simulink model "ADAS_Main_ClosedLoop"  (R2026a)
settings: Solver=FixedStepDiscrete  StopTime=20
InitFcn:
  | createLidarActorProfiles;
  | % L3/L4 closed-loop ego initial condition, READ FROM THE TEST-1 FIXTURE
  | % (not hard-coded in the vehicle model, which stays reusable)
  | clS = load('D:\AutonomousDriving\D_scenarios\V2_0_ClosedLoop_Test9_TwoObstacles_WideRoad.mat');
  | clA = clS.data.ActorSpecifications([clS.data.ActorSpecifications.ActorID] == clS.data.EgoCarId);
  | CL_EGO_IC = [clA.Position(1); clA.Position(2); clA.Yaw*pi/180; clA.Speed(1)];
  | clear clS clA
  | % Non-virtual ego-pose bus type. A MATLAB Function block (Extract_Ego_Kinematics)
  | % cannot accept a VIRTUAL bus, so the Bus Creator must emit a defined Simulink.Bus.
  | % Shape copied from the installed validator contract and from BusActorsActors.
  | clN = {'ActorID','Position','Velocity','Roll','Pitch','Yaw','AngularVelocity'};
  | clD = {[1 1],[1 3],[1 3],[1 1],[1 1],[1 1],[1 3]};
  | clEls = Simulink.BusElement.empty(0,1);
  | for clI = 1:7
  |   clE = Simulink.BusElement; clE.Name = clN{clI}; clE.Dimensions = clD{clI}; clE.DataType = 'double';
  |   clEls(clI,1) = clE;
  | end
  | BusEgoPose_CL = Simulink.Bus; BusEgoPose_CL.Elements = clEls;
  | clear clN clD clEls clE clI
StopFcn:
  | cl_plot_closedloop_trajectory;
model workspace (MAT data in the model file):
  firstWarning = 1
  originalScenarioChecksum = '71EAF3DF157DF5A35F75811B676F8B0F'
undefined symbols (not defined in the file): driving, matlabshared
libraries: drivingscenarioandsensors x3, lidarlib x1
(part 7 of 7)

== matlab function ADAS_Main_ClosedLoop/LiDAR_Perception/LiDAR_Ground_Segmentation/Ground_Height_Model ==
  data: xyzEgo input; groundZ output; groundMask input; groundZValid output
function [groundZ, groundZValid] = Ground_Height_Model(xyzEgo, groundMask)
%#codegen
% GROUND_HEIGHT_MODEL  Compact polar ground-elevation map from LiDAR ground returns.
%
% Inputs
%   xyzEgo     [101 2251 3] double  organized XYZ in the EGO frame
%   groundMask [101 2251]   boolean ground cells from Ground_Segmentation
%                                   (already a subset of the valid mask)
% Outputs
%   groundZ      [72 24] double   ego-frame z of the road surface, metres
%   groundZValid [72 24] boolean  true only where groundZ is a real measurement
%
% COORDINATE FRAME
%   Ego / vehicle frame: origin at the rear-axle centre, X forward, Y left,
%   Z up - the same frame Radar and Vision report in. Cells are indexed by
%   ego-frame polar coordinates about the ego origin:
%       r     = hypot(x,y)          azimuth = atan2(y,x) wrapped to (-pi,pi]
%   so a downstream lookup by an object's own ego-frame range/azimuth is
%   self-consistent with this binning.
%
% BINNING
%   Azimuth: N_AZ uniform sectors over 360 deg.
%   Range:   N_RNG GEOMETRIC (log-spaced) bins over [RMIN, RMAX].
%   Log spacing is dictated by sensor geometry, not by any scenario: the
%   radial gap between consecutive ground hits grows as r^2*dPhi/h, so ground
%   sample density falls as r^2. Uniform rings would put nearly every sample
%   in the first ring. RMAX is the sensor's MaxRange, deliberately NOT tuned
%   to the ground extent of any particular scene; unobserved cells simply
%   report invalid.
%
% ESTIMATION
%   Per cell, the median of stride-sampled ego-frame z values. Stride sampling
%   (rather than first-K) keeps the sample unbiased across the cell instead of
%   favouring one elevation row. The median is robust to the small fraction of
%   mislabelled ground points.
%
% VALIDITY  (groundZValid)
%   1. support : at least MIN_GROUND_PTS_PER_CELL samples in the cell
%   2. flatness: interquartile spread <= MAX_GROUND_SPREAD
%   3. radial slope continuity: walking outward along each azimuth sector, the
%      seed ring must satisfy |z| <= MAX_SLOPE*r + SLOPE_EPS (the ego frame
%      origin sits at ground level, and road grade is physically bounded), and
%      every subsequent accepted ring must be reachable from the previous one
%      at no more than MAX_SLOPE. This rejects flat elevated surfaces - for
%      example a neighbouring vehicle roof - that survive tests 1 and 2.
%
% MISSING REGIONS
%   Where validity fails, groundZ is set to 0 as a NUMERIC PLACEHOLDER ONLY.
%   It is not a measurement and must never be used as one. There is NO
%   interpolation and NO neighbour fallback in this stage: groundZValid means
%   exactly "measured in this cell". Any fallback policy belongs downstream,
%   where it can raise its own observation flag.
%
% SCENARIO INDEPENDENCE
%   Consumes only geometry and the ground mask. No ActorID, ClassID,
%   MaterialID, cluster metadata, actor poses, actor profiles or road geometry.

% ---- parameters: sensor / algorithm / road-physics properties only --------
N_AZ       = 72;      % azimuth sectors (5 deg each)
N_RNG      = 24;      % geometric range bins
RMIN       = 2.0;     % m, inside this lies the ground blind ring
RMAX       = 120.0;   % m, sensor MaxRange
K_SAMPLES  = 32;      % per-cell sample buffer depth
MIN_PTS    = 5;       % minimum support for a trustworthy median
MAX_SPREAD = 0.30;    % m, maximum within-cell interquartile spread
MAX_SLOPE  = 0.20;    % 20 % grade, beyond any drivable road
SLOPE_EPS  = 0.10;    % m, tolerance floor for the slope test

groundZ      = zeros(N_AZ, N_RNG);
groundZValid = false(N_AZ, N_RNG);

count = zeros(N_AZ, N_RNG);
seen  = zeros(N_AZ, N_RNG);
fill  = zeros(N_AZ, N_RNG);
buf   = zeros(N_AZ, N_RNG, K_SAMPLES);

M = size(groundMask, 1);
N = size(groundMask, 2);
logSpan = log(RMAX / RMIN);

% ---- pass 1: count samples per cell ---------------------------------------
for c = 1:N
    for r = 1:M
        if ~groundMask(r, c)
            continue
        end
        x = xyzEgo(r, c, 1);
        y = xyzEgo(r, c, 2);
        rad = hypot(x, y);
        if ~isfinite(rad) || rad < RMIN || rad > RMAX
            continue
        end
        ia = azIndex(y, x, N_AZ);
        ir = rngIndex(rad, RMIN, logSpan, N_RNG);
        count(ia, ir) = count(ia, ir) + 1;
    end
end

% ---- pass 2: stride-sampled fill ------------------------------------------
for c = 1:N
    for r = 1:M
        if ~groundMask(r, c)
            continue
        end
        x = xyzEgo(r, c, 1);
        y = xyzEgo(r, c, 2);
        z = xyzEgo(r, c, 3);
        rad = hypot(x, y);
        if ~isfinite(rad) || rad < RMIN || rad > RMAX || ~isfinite(z)
            continue
        end
        ia = azIndex(y, x, N_AZ);
        ir = rngIndex(rad, RMIN, logSpan, N_RNG);
        seen(ia, ir) = seen(ia, ir) + 1;
        stride = ceil(count(ia, ir) / K_SAMPLES);
        if stride < 1
            stride = 1;
        end
        if mod(seen(ia, ir) - 1, stride) == 0 && fill(ia, ir) < K_SAMPLES
            fill(ia, ir) = fill(ia, ir) + 1;
            buf(ia, ir, fill(ia, ir)) = z;
        end
    end
end

% ---- per-cell median, spread, support/flatness tests ----------------------
rawValid = false(N_AZ, N_RNG);
for ia = 1:N_AZ
    for ir = 1:N_RNG
        m = fill(ia, ir);
        if m < 1
            continue
        end
        % fixed-size buffer; unused slots sort to the end
        v = inf(1, K_SAMPLES);
        for t = 1:K_SAMPLES
            if t <= m
                v(t) = buf(ia, ir, t);
            end
        end
        s = sort(v);

        groundZ(ia, ir) = s(ceil(m / 2));

        if m >= 4
            iLo = max(1, ceil(0.25 * m));
            iHi = ceil(0.75 * m);
            spread = s(iHi) - s(iLo);
        else
            spread = s(m) - s(1);
        end

        rawValid(ia, ir) = (count(ia, ir) >= MIN_PTS) && (spread <= MAX_SPREAD);
    end
end

% ---- radial slope-continuity gate -----------------------------------------
rc = zeros(1, N_RNG);
for ir = 1:N_RNG
    lo = RMIN * exp(logSpan * (ir - 1) / N_RNG);
    hi = RMIN * exp(logSpan * ir / N_RNG);
    rc(ir) = 0.5 * (lo + hi);
end

for ia = 1:N_AZ
    seeded = false;
    zRef = 0;
    rRef = 0;
    for ir = 1:N_RNG
        if ~rawValid(ia, ir)
            continue
        end
        if ~seeded
            if abs(groundZ(ia, ir)) <= MAX_SLOPE * rc(ir) + SLOPE_EPS
                groundZValid(ia, ir) = true;
                seeded = true;
                zRef = groundZ(ia, ir);
                rRef = rc(ir);
            end
        else
            if abs(groundZ(ia, ir) - zRef) <= MAX_SLOPE * abs(rc(ir) - rRef) + SLOPE_EPS
                groundZValid(ia, ir) = true;
                zRef = groundZ(ia, ir);
                rRef = rc(ir);
            end
        end
    end
end

% ---- invalid cells carry no measurement -----------------------------------
for ia = 1:N_AZ
    for ir = 1:N_RNG
        if ~groundZValid(ia, ir)
            groundZ(ia, ir) = 0;
        end
    end
end

end

% ===========================================================================
function ia = azIndex(y, x, N_AZ)
th = atan2(y, x);
ia = floor((th + pi) / (2 * pi) * N_AZ) + 1;
if ia < 1
    ia = 1;
end
if ia > N_AZ
    ia = N_AZ;
end
end

% ===========================================================================
function ir = rngIndex(rad, RMIN, logSpan, N_RNG)
ir = floor(N_RNG * log(rad / RMIN) / logSpan) + 1;
if ir < 1
    ir = 1;
end
if ir > N_RNG
    ir = N_RNG;
end
end

== matlab function ADAS_Main_ClosedLoop/LiDAR_Perception/LiDAR_Clustering/Cluster_BEV ==
  data: xyzEgo input; clusterLabels output; validMask input; groundMask input; numClusters output
function [clusterLabels, numClusters] = Cluster_BEV(xyzEgo, validMask, groundMask)
%#codegen
% CLUSTER_BEV  Bird's-eye-view occupancy clustering of non-ground LiDAR returns.
%
% Inputs
%   xyzEgo     [101 2251 3] double  organized XYZ in the EGO frame
%   validMask  [101 2251]   boolean finite, non-ego points
%   groundMask [101 2251]   boolean ground points (excluded from clustering)
% Outputs
%   clusterLabels [101 2251] uint32  0 = unclustered, else 1..numClusters
%   numClusters   scalar     uint32  number of surviving clusters
%
% METHOD
%   Non-ground valid points are projected onto a Cartesian BEV occupancy grid
%   and grouped with 8-connected components (two-pass Rosenfeld + union-find).
%   Chosen over organized range-image clustering (segmentLidarData) and
%   Euclidean kd-tree clustering (pcsegdist) after measuring all three on 51
%   frames: the range-image method fragmented badly and could not be tuned out
%   of it - ground removal punches NaN holes through the range image that
%   disconnect object pixels - and the kd-tree method cost ~25x more for no
%   quality gain. A 0.30 m cell preserves more VRU-scale objects AND over-merges
%   less than coarser cells.
%
% DETERMINISM
%   Raster scan order is fixed, unions always point to the smaller root, and
%   final IDs are assigned in ascending root order. Identical input gives
%   identical output.
%
% SCENARIO INDEPENDENCE
%   Consumes only geometry and the two masks. No actor identity, no class, no
%   material, no cluster metadata, no actor poses or profiles, no scenario
%   geometry, no ground-height model. No velocity or behaviour is estimated.

% ---- parameters (sensor / algorithm properties) ---------------------------
CELL_SIZE  = 0.30;      % m, BEV cell edge
GRID_LIM   = 120.0;     % m, half-extent = sensor MaxRange
GRID_N     = 802;       % cells per axis: floor(2*120/0.30)+1 = 801, +1 margin
MIN_PTS    = 10;        % minimum points for a cluster to survive
MAX_CLUST  = 256;       % fixed capacity of the cluster interface
MAX_LABELS = 131072;    % provisional-label capacity (measured peak: 945)

M = size(validMask, 1);
N = size(validMask, 2);

clusterLabels = zeros(M, N, 'uint32');
numClusters   = uint32(0);

occ     = false(GRID_N, GRID_N);
cellLab = zeros(GRID_N, GRID_N, 'uint32');
parent  = zeros(MAX_LABELS, 1, 'uint32');
compPts = zeros(MAX_LABELS, 1, 'uint32');
finalId = zeros(MAX_LABELS, 1, 'uint32');

% Hoist the two channels into contiguous 2-D planes. Indexing xyzEgo(r,c,1)
% and (r,c,2) directly costs a stride of M*N elements between the two reads,
% which thrashes the cache across three passes over 227k points.
X = xyzEgo(:, :, 1);
Y = xyzEgo(:, :, 2);

% Per-point BEV cell, computed once and reused by the later passes.
cellIdx = zeros(M, N, 'int32');

% ---- pass A: eligibility, cell index, occupancy ---------------------------
minIx = GRID_N; maxIx = 1; minIy = GRID_N; maxIy = 1; anyOcc = false;
for c = 1:N
    for r = 1:M
        if ~validMask(r, c) || groundMask(r, c)
            continue
        end
        x = X(r, c);
        y = Y(r, c);
        if ~isfinite(x) || ~isfinite(y)
            continue
        end
        if x < -GRID_LIM || x > GRID_LIM || y < -GRID_LIM || y > GRID_LIM
            continue                        % outside the grid: never clustered
        end
        ix = floor((x + GRID_LIM) / CELL_SIZE) + 1;
        iy = floor((y + GRID_LIM) / CELL_SIZE) + 1;
        if ix < 1,      ix = 1;      end
        if ix > GRID_N, ix = GRID_N; end
        if iy < 1,      iy = 1;      end
        if iy > GRID_N, iy = GRID_N; end
        occ(ix, iy) = true;
        cellIdx(r, c) = int32((iy - 1) * GRID_N + ix);
        anyOcc = true;
        if ix < minIx, minIx = ix; end
        if ix > maxIx, maxIx = ix; end
        if iy < minIy, minIy = iy; end
        if iy > maxIy, maxIy = iy; end
    end
end

if ~anyOcc
    return
end

% ---- pass B: provisional labels with inline union-find --------------------
% Only the occupied bounding box is scanned. Cells outside it are empty by
% construction, so this is an exact optimisation, not an approximation.
nLab = 0;
for iy = minIy:maxIy
    for ix = minIx:maxIx
        if ~occ(ix, iy)
            continue
        end

        % the four already-scanned 8-neighbours: W, NW, N, NE
        nb = zeros(1, 4);
        if ix > 1,                nb(1) = double(cellLab(ix-1, iy  )); end
        if ix > 1  && iy > 1,     nb(2) = double(cellLab(ix-1, iy-1)); end
        if iy > 1,                nb(3) = double(cellLab(ix  , iy-1)); end
        if ix < GRID_N && iy > 1, nb(4) = double(cellLab(ix+1, iy-1)); end

        mn = 0;
        for k = 1:4
            if nb(k) > 0
                rk = nb(k);
                while double(parent(rk)) ~= rk
                    rk = double(parent(rk));
                end
                if mn == 0 || rk < mn
                    mn = rk;
                end
            end
        end

        if mn == 0
            if nLab < MAX_LABELS
                nLab = nLab + 1;
                parent(nLab) = uint32(nLab);
                cellLab(ix, iy) = uint32(nLab);
            end
            % label space exhausted: cell stays 0 and is simply not clustered
        else
            cellLab(ix, iy) = uint32(mn);
            for k = 1:4
                if nb(k) > 0
                    ra = nb(k);
                    while double(parent(ra)) ~= ra
                        ra = double(parent(ra));
                    end
                    if ra ~= mn
                        if ra < mn
                            parent(mn) = uint32(ra);
                            mn = ra;
                        else
                            parent(ra) = uint32(mn);
                        end
                    end
                end
            end
        end
    end
end

% ---- flatten: unions always point to a smaller index, so one pass suffices -
for k = 1:nLab
    p = double(parent(k));
    if p ~= k
        parent(k) = parent(p);
    end
end

% ---- pass C: count points per component -----------------------------------
for c = 1:N
    for r = 1:M
        ci = double(cellIdx(r, c));
        if ci <= 0
            continue
        end
        lb = double(cellLab(ci));
        if lb > 0
            rt = double(parent(lb));
            compPts(rt) = compPts(rt) + uint32(1);
        end
    end
end

% ---- select surviving components ------------------------------------------
nSurv = 0;
survRoot = zeros(MAX_LABELS, 1, 'uint32');
for k = 1:nLab
    if double(parent(k)) == k && compPts(k) >= uint32(MIN_PTS)
        nSurv = nSurv + 1;
        survRoot(nSurv) = uint32(k);
    end
end

keepFlag = false(MAX_LABELS, 1);
if nSurv <= MAX_CLUST
    for s = 1:nSurv
        keepFlag(double(survRoot(s))) = true;
    end
else
    % over capacity: keep the MAX_CLUST largest, tie-break on lower root index
    taken = false(MAX_LABELS, 1);
    for t = 1:MAX_CLUST
        bestIdx = 0;
        bestCnt = uint32(0);
        for s = 1:nSurv
            rt = double(survRoot(s));
            if taken(rt)
                continue
            end
            if bestIdx == 0 || compPts(rt) > bestCnt
                bestIdx = rt;
                bestCnt = compPts(rt);
            end
        end
        if bestIdx == 0
            break
        end
        taken(bestIdx)    = true;
        keepFlag(bestIdx) = true;
    end
end

% final IDs in ascending root order, so labels are stable across frames
nid = 0;
for k = 1:nLab
    if keepFlag(k)
        nid = nid + 1;
        finalId(k) = uint32(nid);
    end
end
numClusters = uint32(nid);

% ---- pass D: map labels back onto the organized grid ----------------------
for c = 1:N
    for r = 1:M
        ci = double(cellIdx(r, c));
        if ci <= 0
            continue
        end
        lb = double(cellLab(ci));
        if lb > 0
            clusterLabels(r, c) = finalId(double(parent(lb)));
        end
    end
end

end

== matlab function ADAS_Main_ClosedLoop/LiDAR_Perception/LiDAR_Object_Features/Extract_Object_Features ==
  data: xyzEgo input; LiDARFeatures output; intensityIn input; validMask input; groundMask input; groundZ input; groundZValid input; clusterLabels input; numClusters input
function LiDARFeatures = Extract_Object_Features(xyzEgo, intensityIn, validMask, ...
    groundMask, groundZ, groundZValid, clusterLabels, numClusters)
%#codegen
% EXTRACT_OBJECT_FEATURES  Object-level features for up to 256 LiDAR clusters.
%
% Output: LiDARFeatures [256 x 20] double, ego frame throughout.
%   1  Valid              0/1
%   2  PosX               m    centroid (mean) x
%   3  PosY               m    centroid y
%   4  PosZ               m    centroid z   (kept: not derivable from ZBottom+Height)
%   5  CovXX              m^2  position uncertainty
%   6  CovYY              m^2
%   7  CovXY              m^2  cross term: the error ellipse aligns to the line of
%                              sight, not the ego axes
%   8  CovZZ              m^2
%   9  Length             m    oriented (PCA) extent along the principal axis
%   10 Width              m    oriented extent across it
%   11 Height             m    zmax - zmin
%   12 Yaw                rad  principal-axis direction
%   13 ZBottom            m    min z
%   14 HeightAboveGround  m    ZBottom - ground; MEANINGLESS unless bit 64 is clear
%   15 ClosestX           m    nearest point of the cluster (TTC geometry)
%   16 ClosestY           m
%   17 PointCount         -
%   18 IntensityMean      0-255  association/measurement evidence ONLY, never a class cue
%   19 Confidence         0-1  geometric detectability
%   20 ObservationFlags   bitfield, see below
%
% ObservationFlags
%   1   Sparse            n < SPARSE_N
%   2   DegenerateShape   eigenvalue ratio < DEGEN_RATIO (1-D scatter)
%   4   ThinFootprint     oriented width < one BEV cell
%   8   ExtentUntrusted   any of 1/2/4 - Length/Width/Height/Yaw are not measurements
%   16  YawAmbiguous      eigenvalue ratio > AMBIG_RATIO (near-circular)
%   32  AzimuthSeam       cluster straddles +/-180 deg
%   64  GroundUnavailable no ground reference; HeightAboveGround is a placeholder 0
%   128 GroundInferred    ground taken from a bounded neighbour, not this cell
%   256 ElevFovEdge       touches the top or bottom elevation row
%   512 RangeTruncated    nearest point beyond TRUNC_RANGE
%
% SCENARIO INDEPENDENCE
%   Consumes only geometry, intensity and the validated masks/labels. No ActorID,
%   ClassID, MaterialID, cluster metadata, actor poses, actor profiles or
%   scenario geometry. No velocity or behaviour is estimated here.

MAXC = 256;
NCOL = 20;

% sensor / algorithm constants
AZ_RES      = 0.16 * pi/180;   % rad, azimuth resolution
EL_RES      = 0.40 * pi/180;   % rad, elevation resolution
SIGMA_R     = 0.01;            % m, sensor RangeAccuracy
NEFF_CAP    = 25;              % correlated returns on one surface
SPARSE_N    = 30;
DEGEN_RATIO = 0.05;
AMBIG_RATIO = 0.80;
CELL_SIZE   = 0.30;            % m, BEV cell used by the clustering stage
TRUNC_RANGE = 118.0;           % m
A_REF       = 1.5;             % m^2, nominal visible face for the confidence model
R_REF       = 20.0;            % m
SIG_MIN     = 0.10;            % m
SIG_MAX     = 2.00;            % m
GAMMA_ALONG = 0.25;            % unobserved-depth bias
GAMMA_CROSS = 0.12;

LiDARFeatures = zeros(MAXC, NCOL);

K = double(numClusters);
if K < 1
    return
end
if K > MAXC
    K = MAXC;
end

M = size(validMask, 1);
N = size(validMask, 2);

% Hoist the planes: indexing xyzEgo(r,c,1..3) directly costs a stride of M*N
% elements between channel reads, across two passes over 227k points.
X = xyzEgo(:, :, 1);
Y = xyzEgo(:, :, 2);
Z = xyzEgo(:, :, 3);

n   = zeros(MAXC,1); sx = zeros(MAXC,1); sy = zeros(MAXC,1); sz = zeros(MAXC,1);
sxx = zeros(MAXC,1); syy = zeros(MAXC,1); sxy = zeros(MAXC,1); si = zeros(MAXC,1);
xmn = inf(MAXC,1); xmx = -inf(MAXC,1);
ymn = inf(MAXC,1); ymx = -inf(MAXC,1);
zmn = inf(MAXC,1); zmx = -inf(MAXC,1);
rmn = inf(MAXC,1); clx = zeros(MAXC,1); cly = zeros(MAXC,1);
rowMin = inf(MAXC,1); rowMax = -inf(MAXC,1);
azMin  = inf(MAXC,1); azMax  = -inf(MAXC,1);

% ---- pass 1: moments, extremes, closest point -----------------------------
for c = 1:N
    for r = 1:M
        k = double(clusterLabels(r, c));
        if k < 1 || k > K
            continue
        end
        % guard: a labelled point must also be valid and non-ground
        if ~validMask(r, c) || groundMask(r, c)
            continue
        end
        x = X(r, c); y = Y(r, c); z = Z(r, c);
        n(k)   = n(k) + 1;
        sx(k)  = sx(k) + x;   sy(k)  = sy(k) + y;   sz(k) = sz(k) + z;
        sxx(k) = sxx(k) + x*x;
        syy(k) = syy(k) + y*y;
        sxy(k) = sxy(k) + x*y;
        si(k)  = si(k) + double(intensityIn(r, c));
        if x < xmn(k), xmn(k) = x; end
        if x > xmx(k), xmx(k) = x; end
        if y < ymn(k), ymn(k) = y; end
        if y > ymx(k), ymx(k) = y; end
        if z < zmn(k), zmn(k) = z; end
        if z > zmx(k), zmx(k) = z; end
        rr = hypot(x, y);
        if rr < rmn(k)
            rmn(k) = rr; clx(k) = x; cly(k) = y;
        end
        if r < rowMin(k), rowMin(k) = r; end
        if r > rowMax(k), rowMax(k) = r; end
        a = atan2(y, x);
        if a < azMin(k), azMin(k) = a; end
        if a > azMax(k), azMax(k) = a; end
    end
end

% ---- principal axes from the accumulated moments --------------------------
yaw  = zeros(MAXC,1);
evR  = zeros(MAXC,1);
for k = 1:K
    if n(k) < 2
        continue
    end
    mx = sx(k)/n(k); my = sy(k)/n(k);
    cxx = sxx(k)/n(k) - mx*mx;
    cyy = syy(k)/n(k) - my*my;
    cxy = sxy(k)/n(k) - mx*my;
    tr = cxx + cyy;
    dt = cxx*cyy - cxy*cxy;
    disc = tr*tr/4 - dt;
    if disc < 0
        disc = 0;
    end
    l1 = tr/2 + sqrt(disc);
    l2 = tr/2 - sqrt(disc);
    if abs(cxy) > 1e-12
        yaw(k) = atan2(l1 - cxx, cxy);
    elseif cxx >= cyy
        yaw(k) = 0;
    else
        yaw(k) = pi/2;
    end
    if l1 > 0
        if l2 < 0
            evR(k) = 0;
        else
            evR(k) = l2/l1;
        end
    end
end

% ---- pass 2: oriented extents ---------------------------------------------
p1mn = inf(MAXC,1); p1mx = -inf(MAXC,1);
p2mn = inf(MAXC,1); p2mx = -inf(MAXC,1);
for c = 1:N
    for r = 1:M
        k = double(clusterLabels(r, c));
        if k < 1 || k > K
            continue
        end
        if ~validMask(r, c) || groundMask(r, c)
            continue
        end
        dx = X(r, c) - sx(k)/n(k);
        dy = Y(r, c) - sy(k)/n(k);
        ca = cos(yaw(k)); sa = sin(yaw(k));
        p1 =  dx*ca + dy*sa;
        p2 = -dx*sa + dy*ca;
        if p1 < p1mn(k), p1mn(k) = p1; end
        if p1 > p1mx(k), p1mx(k) = p1; end
        if p2 < p2mn(k), p2mn(k) = p2; end
        if p2 > p2mx(k), p2mx(k) = p2; end
    end
end

N_REF = A_REF/(R_REF*R_REF*AZ_RES*EL_RES);

% ---- finalise -------------------------------------------------------------
for k = 1:K
    if n(k) < 1
        continue
    end
    cx = sx(k)/n(k);
    cy = sy(k)/n(k);
    cz = sz(k)/n(k);
    Lq = p1mx(k) - p1mn(k);
    Wq = p2mx(k) - p2mn(k);
    Hq = zmx(k) - zmn(k);
    rng = hypot(cx, cy);
    az  = atan2(cy, cx);

    % ---- ground reference: direct cell first, bounded neighbour only if it fails
    [gv, gOK, gInferred] = groundRef(cx, cy, groundZ, groundZValid);
    if gOK
        hag = zmn(k) - gv;
    else
        hag = 0;                 % placeholder only; bit 64 marks it as meaningless
    end

    % ---- flags
    fg = 0;
    if n(k) < SPARSE_N,      fg = fg + 1;   end
    if evR(k) < DEGEN_RATIO, fg = fg + 2;   end
    if Wq < CELL_SIZE,       fg = fg + 4;   end
    if fg > 0,               fg = fg + 8;   end
    if evR(k) > AMBIG_RATIO, fg = fg + 16;  end
    if (azMax(k) - azMin(k)) > pi, fg = fg + 32; end
    if ~gOK,                 fg = fg + 64;  end
    if gInferred,            fg = fg + 128; end
    if rowMin(k) <= 2 || rowMax(k) >= M-1,  fg = fg + 256; end
    if rmn(k) > TRUNC_RANGE, fg = fg + 512; end

    % ---- position uncertainty
    sAz  = rng*AZ_RES/sqrt(12);
    sEl  = rng*EL_RES/sqrt(12);
    nEff = n(k);
    if nEff > NEFF_CAP
        nEff = NEFF_CAP;
    end
    dAng  = yaw(k) - az;
    extA  = abs(Lq*cos(dAng)) + abs(Wq*sin(dAng));
    extC  = abs(Lq*sin(dAng)) + abs(Wq*cos(dAng));
    if extA < 0.1, extA = 0.1; end
    if extC < 0.1, extC = 0.1; end
    sAlong = sqrt((SIGMA_R/sqrt(nEff))^2 + (GAMMA_ALONG*extA)^2);
    sCross = sqrt((sAz/sqrt(nEff))^2     + (GAMMA_CROSS*extC)^2);
    if sAlong < SIG_MIN, sAlong = SIG_MIN; end
    if sAlong > SIG_MAX, sAlong = SIG_MAX; end
    if sCross < SIG_MIN, sCross = SIG_MIN; end
    if sCross > SIG_MAX, sCross = SIG_MAX; end
    ca = cos(az); sa = sin(az);
    covXX = sAlong*sAlong*ca*ca + sCross*sCross*sa*sa;
    covYY = sAlong*sAlong*sa*sa + sCross*sCross*ca*ca;
    covXY = (sAlong*sAlong - sCross*sCross)*ca*sa;
    covZZ = (sEl/sqrt(nEff))^2 + (0.10*Hq)^2;
    if covZZ < 0.05^2
        covZZ = 0.05^2;
    end

    % ---- confidence: fixed sensor geometry, NOT the measured angular span
    rClamp = rng;
    if rClamp < 1, rClamp = 1; end
    nExp = N_REF*(R_REF/rClamp)^2;
    if nExp < 1, nExp = 1; end
    conf = n(k)/nExp;
    if conf > 1, conf = 1; end
    if rowMin(k) <= 2 || rowMax(k) >= M-1 || rmn(k) > TRUNC_RANGE
        conf = conf*0.7;
    end

    LiDARFeatures(k, 1)  = 1;
    LiDARFeatures(k, 2)  = cx;
    LiDARFeatures(k, 3)  = cy;
    LiDARFeatures(k, 4)  = cz;
    LiDARFeatures(k, 5)  = covXX;
    LiDARFeatures(k, 6)  = covYY;
    LiDARFeatures(k, 7)  = covXY;
    LiDARFeatures(k, 8)  = covZZ;
    LiDARFeatures(k, 9)  = Lq;
    LiDARFeatures(k, 10) = Wq;
    LiDARFeatures(k, 11) = Hq;
    LiDARFeatures(k, 12) = yaw(k);
    LiDARFeatures(k, 13) = zmn(k);
    LiDARFeatures(k, 14) = hag;
    LiDARFeatures(k, 15) = clx(k);
    LiDARFeatures(k, 16) = cly(k);
    LiDARFeatures(k, 17) = n(k);
    LiDARFeatures(k, 18) = si(k)/n(k);
    LiDARFeatures(k, 19) = conf;
    LiDARFeatures(k, 20) = fg;
end

end

% ===========================================================================
function [g, ok, inferred] = groundRef(x, y, groundZ, groundZValid)
% Direct cell lookup first. A directly valid measurement is returned before any
% neighbour is examined, so it can never be overwritten by a neighbour value.
N_AZ = 72; N_RNG = 24; RMIN = 2.0; RMAX = 120.0;
g = 0; ok = false; inferred = false;

r = hypot(x, y);
if ~isfinite(r) || r < RMIN || r > RMAX
    return
end
Lg = log(RMAX/RMIN);
th = atan2(y, x);
a = floor((th + pi)/(2*pi)*N_AZ) + 1;
if a < 1, a = 1; end
if a > N_AZ, a = N_AZ; end
b = floor(N_RNG*log(r/RMIN)/Lg) + 1;
if b < 1, b = 1; end
if b > N_RNG, b = N_RNG; end

if groundZValid(a, b)
    g = groundZ(a, b);
    ok = true;
    return                      % direct measurement wins outright
end

% bounded neighbourhood: +/-2 azimuth sectors in the same range ring
for da = -2:2
    aa = mod(a - 1 + da, N_AZ) + 1;
    if groundZValid(aa, b)
        g = groundZ(aa, b);
        ok = true;
        inferred = true;
        return
    end
end
% then +/-1 range ring in the same sector
for db = -1:2:1
    bb = b + db;
    if bb >= 1 && bb <= N_RNG
        if groundZValid(a, bb)
            g = groundZ(a, bb);
            ok = true;
            inferred = true;
            return
        end
    end
end
end

== matlab function ADAS_Main_ClosedLoop/LiDAR_Perception/LiDAR_Detection_Formatting/Format_LiDAR_Detections ==
  data: LiDARFeatures input; LiDARDetections output; numClusters input; NumLiDARDetections output
function [LiDARDetections, NumLiDARDetections] = Format_LiDAR_Detections(LiDARFeatures, numClusters)
%#codegen
% FORMAT_LIDAR_DETECTIONS  Final fixed-size LiDAR detection interface.
%
% Inputs
%   LiDARFeatures [256 x 20] double  validated object features
%   numClusters   scalar    uint32   number of populated feature rows
% Outputs
%   LiDARDetections    [256 x 20] double  ranked, filtered, zero-padded
%   NumLiDARDetections scalar    uint32  count of valid output rows
%
% This stage performs ONLY selection, ranking, truncation and interface
% formatting. It does not classify, does not estimate velocity, and does not
% infer intent. Its only inputs are the feature matrix and the cluster count,
% so it structurally cannot reach ActorID, ClassID, MaterialID, cluster
% metadata, actor poses, actor profiles or scenario geometry.
%
% CANDIDATE FILTERING - exactly three physical rules, never a flag:
%   A  ground available AND HeightAboveGround >  2.5 m   (overhead structure)
%   B  ground available AND HeightAboveGround < -0.5 m   (below-ground artefact)
%   C  Confidence < 0.02                                 (negligible evidence)
%
% Candidates are NEVER discarded for Sparse, DegenerateShape, ThinFootprint,
% ExtentUntrusted, GroundUnavailable, GroundInferred, YawAmbiguous,
% AzimuthSeam, ElevFovEdge or RangeTruncated. Measured on 51 frames, filtering
% on ExtentUntrusted alone would have deleted 96.8% of small near candidates -
% the pedestrians, bicycles and two-wheelers this system exists to protect.
% A geometrically weak cluster is not an invalid detection: its position and
% covariance remain useful to Sensor Fusion and Tracking.
%
% Geometric values are preserved even when ExtentUntrusted is set. They are NOT
% zeroed: zeroing would make "unknown" indistinguishable from "measured zero",
% and the footprint is still a genuine lower bound on extent.
%
% ObservationFlags pass through bit-for-bit (whole rows are copied verbatim).
%
% RANKING
%   Ascending hypot(ClosestX, ClosestY), so truncation always sheds the
%   farthest - least safety-critical - candidates first. The sort is stable,
%   so equal ranges keep the lower original feature-row index.

MAX_IN   = 256;
MAX_OUT  = 256;
NCOL     = 20;

% column indices in LiDARFeatures
C_VALID  = 1;
C_HAG    = 14;
C_CLX    = 15;
C_CLY    = 16;
C_CONF   = 19;
C_FLAGS  = 20;

% filter thresholds
HAG_MAX      = 2.5;    % m, above this the cluster is overhead structure
HAG_MIN      = -0.5;   % m, below this it is a below-ground artefact
CONF_MIN     = 0.02;   % negligible evidence
FLAG_NOGND   = uint32(64);

LiDARDetections    = zeros(MAX_OUT, NCOL);
NumLiDARDetections = uint32(0);

K = double(numClusters);
if K < 1
    return
end
if K > MAX_IN
    K = MAX_IN;
end

survIdx = zeros(MAX_IN, 1);
survRng = zeros(MAX_IN, 1);
nSurv   = 0;

% ---- filter, collecting survivors in ascending feature-row order ----------
for i = 1:K
    if LiDARFeatures(i, C_VALID) ~= 1
        continue
    end

    flags = uint32(LiDARFeatures(i, C_FLAGS));
    groundAvailable = bitand(flags, FLAG_NOGND) == 0;
    hag  = LiDARFeatures(i, C_HAG);
    conf = LiDARFeatures(i, C_CONF);

    ruleA = groundAvailable && (hag > HAG_MAX);
    ruleB = groundAvailable && (hag < HAG_MIN);
    ruleC = conf < CONF_MIN;

    if ruleA || ruleB || ruleC
        continue
    end

    nSurv = nSurv + 1;
    survIdx(nSurv) = i;
    survRng(nSurv) = hypot(LiDARFeatures(i, C_CLX), LiDARFeatures(i, C_CLY));
end

if nSurv < 1
    return
end

% ---- stable insertion sort on range --------------------------------------
% Strict '>' keeps equal ranges in their original (ascending index) order,
% which is the specified deterministic tie-break.
for a = 2:nSurv
    keyR = survRng(a);
    keyI = survIdx(a);
    b = a - 1;
    while b >= 1 && survRng(b) > keyR
        survRng(b+1) = survRng(b);
        survIdx(b+1) = survIdx(b);
        b = b - 1;
    end
    survRng(b+1) = keyR;
    survIdx(b+1) = keyI;
end

% ---- truncate to capacity, copy whole rows verbatim ----------------------
nOut = nSurv;
if nOut > MAX_OUT
    nOut = MAX_OUT;
end

for j = 1:nOut
    src = survIdx(j);
    for c = 1:NCOL
        LiDARDetections(j, c) = LiDARFeatures(src, c);
    end
end

NumLiDARDetections = uint32(nOut);

end
